simulink model "lab4_simulink4"  (R2024a)
settings: Solver=VariableStepAuto  StartTime=0.0  StopTime=10.0  RelTol=1e-3
values from neighbouring files (symbols this model uses):
  C = 1*u    (= 1e-06)    [project1.m]
undefined symbols (not defined in the file or in its folder): designMultirateFIR
libraries: dspmlti4 x3, dspfdesign x2, dspsnks4 x1, dspvision x1
settings Model: Creator=PULLEY  LastModifiedBy=PULLEY

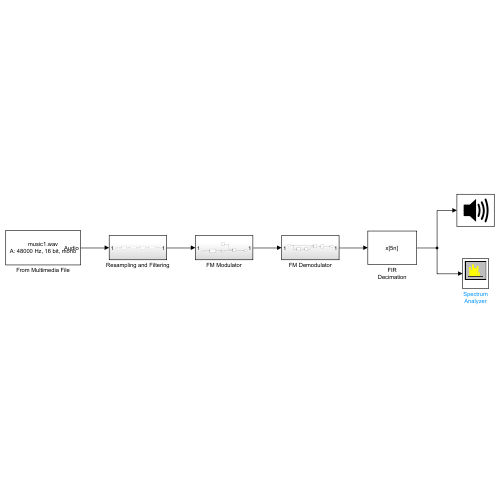
[thumbnail: Simulink's stored preview of the top-level diagram]
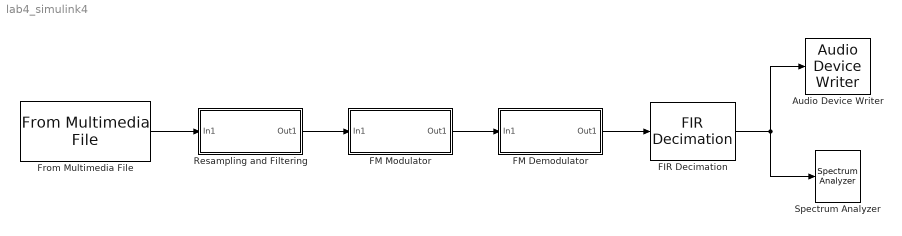
== system lab4_simulink4 ==
  Audio Device Writer : dspsnks4/Audio Device Writer  Driver=DirectSound  Device=Default  InheritSampleRate=on  SampleRate=44100  BitDepth=16-bit integer  BufferSize=4096  NumBuffers=10  DefaultOutputChannelMapping=on  OutputChannelMapping=1:2  OutputNumUnderrunSamples=off  DriverIdx=1  DeviceWarnFlag=''
  FIR Decimation : dspmlti4/FIR Decimation  FilterSource=Auto  h=designMultirateFIR(1,2)  D=5  filtStruct=Direct form  FilterObject=FDECIM  InputProcessing=Columns as channels (frame based)  framing=Enforce single-rate processing  AllowArbitraryInputLength=off  inputOffset=0  outputBufInitCond=0  roundingMode=Floor  overflowMode=off  firstCoeffDataTypeStr=Inherit: Same word length as input  firstCoeffMin=[]  firstCoeffMax=[]  firstCoeffLastDataTypeStr=Inherit: Same word length as input  outputDataTypeStr=Inherit: Same as accumulator  outputMin=[]  outputMax=[]  outputLastDataTypeStr=Inherit: Same as accumulator
      settings: LibrarySourceBlock=|
      | dsphdlsupportfiltering/FIR
      | Decimation
  FM Demodulator : Subsystem
  FM Modulator : Subsystem
  From Multimedia File : dspvision/From Multimedia File  inputFilename=C:\Users\pulley\Downloads\music1.wav  readRange=[1 Inf]  loop=on  numPlays=inf  outputStreams=Audio only  videoDataType=single  audioDataType=double  inheritSampleTime=on  userDefinedSampleTime=1/30  noAudioOutput=off  isIntensityVideo=off  fourcc=RGB  colorVideoFormat=One multidimensional signal  outputEOF=off  dataOrg=Column-major  audioFrameSize=1024  computeAudioFrameSize=off  outSamplingMode=Sample based
      settings: LibrarySourceBlock=dspsrcs4/From Multimedia File
  Resampling and Filtering : Subsystem
  Spectrum Analyzer : SpectrumAnalyzer  WindowPosition=[440.000000,275.000000,800.000000,500.000000,]  Visible=on  ScopeFrameLocation=window  ExpandToolstrip=on  SelectedToolstripTab=spectrumAnalyzerToolstrip.channelMeasurementsTab
  wires:
  From Multimedia File/1 -> Resampling and Filtering/1(In1)
  Resampling and Filtering/1(Out1) -> FM Modulator/1(In1)
  FM Modulator/1(Out1) -> FM Demodulator/1(In1)
  FM Demodulator/1(Out1) -> FIR Decimation/1
  FIR Decimation/1 -> Spectrum Analyzer/1, Audio Device Writer/1

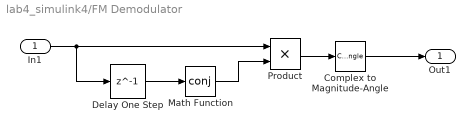
== system lab4_simulink4/FM Demodulator ==
  In1 : Inport
  Complex to Magnitude-Angle : ComplexToMagnitudeAngle  Output=Angle
  Delay One Step : Delay  DelayLength=1
  Math Function : Math  Operator=conj
  Product : Product
  Out1 : Outport
  wires:
  Delay One Step/1 -> Math Function/1
  Math Function/1 -> Product/2
  In1/1 -> Delay One Step/1, Product/1
  Product/1 -> Complex to Magnitude-Angle/1
  Complex to Magnitude-Angle/1 -> Out1/1

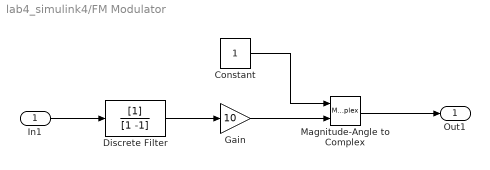
== system lab4_simulink4/FM Modulator ==
  In1 : Inport
  Constant : Constant
  Discrete Filter : DiscreteFilter  Denominator=[1 -1]
  Gain : Gain  Gain=10
  Magnitude-Angle to Complex : MagnitudeAngleToComplex
  Out1 : Outport
  wires:
  In1/1 -> Discrete Filter/1
  Discrete Filter/1 -> Gain/1
  Gain/1 -> Magnitude-Angle to Complex/2
  Constant/1 -> Magnitude-Angle to Complex/1
  Magnitude-Angle to Complex/1 -> Out1/1

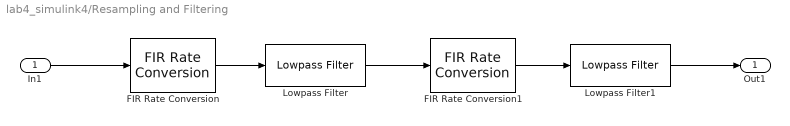
== system lab4_simulink4/Resampling and Filtering ==
  In1 : Inport
  FIR Rate Conversion : dspmlti4/FIR Rate Conversion  FilterSource=Auto  L=5  h=designMultirateFIR(3,2)  M=2  FilterObject=FRC  rateMode=Enforce single-rate processing  AllowArbitraryInputLength=off  roundingMode=Floor  overflowMode=off  firstCoeffDataTypeStr=Inherit: Same word length as input  firstCoeffMin=[]  firstCoeffMax=[]  firstCoeffLastDataTypeStr=Inherit: Same word length as input  outputDataTypeStr=Inherit: Same as accumulator  outputMin=[]  outputMax=[]  outputLastDataTypeStr=Inherit: Same as accumulator
  FIR Rate Conversion1 : dspmlti4/FIR Rate Conversion  FilterSource=Auto  L=5  h=designMultirateFIR(3,2)  M=3  FilterObject=FRC  rateMode=Enforce single-rate processing  AllowArbitraryInputLength=off  roundingMode=Floor  overflowMode=off  firstCoeffDataTypeStr=Inherit: Same word length as input  firstCoeffMin=[]  firstCoeffMax=[]  firstCoeffLastDataTypeStr=Inherit: Same word length as input  outputDataTypeStr=Inherit: Same as accumulator  outputMin=[]  outputMax=[]  outputLastDataTypeStr=Inherit: Same as accumulator
  Lowpass Filter : dspfdesign/Lowpass Filter  FilterType=FIR  DesignForMinimumOrder=on  FilterOrder=50  PassbandFrequency=15e3  StopbandFrequency=24e3  PassbandRipple=0.1  StopbandAttenuation=80  SampleRate=44100  SimulateUsing=Interpreted execution  roundingMode=Floor  coeffsDataTypeStr=fixdt(1,16)
  Lowpass Filter1 : dspfdesign/Lowpass Filter  FilterType=FIR  DesignForMinimumOrder=on  FilterOrder=50  PassbandFrequency=15e3  StopbandFrequency=24e3  PassbandRipple=0.1  StopbandAttenuation=80  SampleRate=44100  SimulateUsing=Interpreted execution  roundingMode=Floor  coeffsDataTypeStr=fixdt(1,16)
  Out1 : Outport
  wires:
  In1/1 -> FIR Rate Conversion/1
  FIR Rate Conversion/1 -> Lowpass Filter/1
  Lowpass Filter/1 -> FIR Rate Conversion1/1
  FIR Rate Conversion1/1 -> Lowpass Filter1/1
  Lowpass Filter1/1 -> Out1/1
